simulink model "Current_Fed_DC_DC_Converter_Code_Equivalent_v4"  (R2020a)
settings: Solver=ode3  StartTime=0.0  StopTime=0.4  MaxStep=1e-5  MinStep=1e-7  RelTol=1e-6
InitFcn:
  | %Supply
  | V_supply = 415;
  | f_supply = 50;
  | 
  | %DC_Bus
  | C_filt = 220e-6
  | L_dc = 100e-6;
  | C_out = 560e-3;
  | 
  | %Transformer
  | P_TX = 10e3;
  | V_pri = 36;
  | V_sec = 1;
  | L_leak = 0;
  | R_leak = 0;
  | L_mag = inf;
  | R_mag = inf;
  | 
  | %Control
  | f_sw = 15e3;
  | tss_conv = 0.1;
  | V_ref = 1480;
  | Kp_V = 1;
  | Ki_V = 0.001;
  | I_ref = 2920;
  | Kp_I = 0.025;
  | Ki_I = 0.000001;
  | PS_max = 180;
  | Carr_offset = 1;
  | Carr_scale = 0.5;
  | Duty_scale = 0.01;
  | Duty_fix = 50;
  | Duty_max = 75;
  | Duty_min = 0;
  | f_chop = 1e3;
  | Duty_chop = 40;
  | 
  | %Harmonic_Correction
  | P_inj = 50;
  | f_inj = 50;
  | L_inj = 10e-6;
  | R_inj = 1;
  | Vpri_inj = 1;
  | Vsec_inj = 70;
  | Rleak_inj = 1e-3;
  | Lleak_inj = 12e-6;
  | R_inj = 0.1;
  | Rmag_inj = 1e-3;
  | Lmag_inj = 1e-3;
  | 
  | %Sensor
  | ADC_Res = 4096;
  | I_sense = 1/700;
  | V_sense = 1/50;
  | 
  | %Faults
  | OV_limit = 18.25;
  | UV_limit = 17.5;
  | OC_limit = 515;
  | UC_limit = 22;
  | ... (+3 lines)
libraries: powerlib x109, powerlib_meascontrol x30, simulink x5, slctrlblks x2
(part 3 of 3)

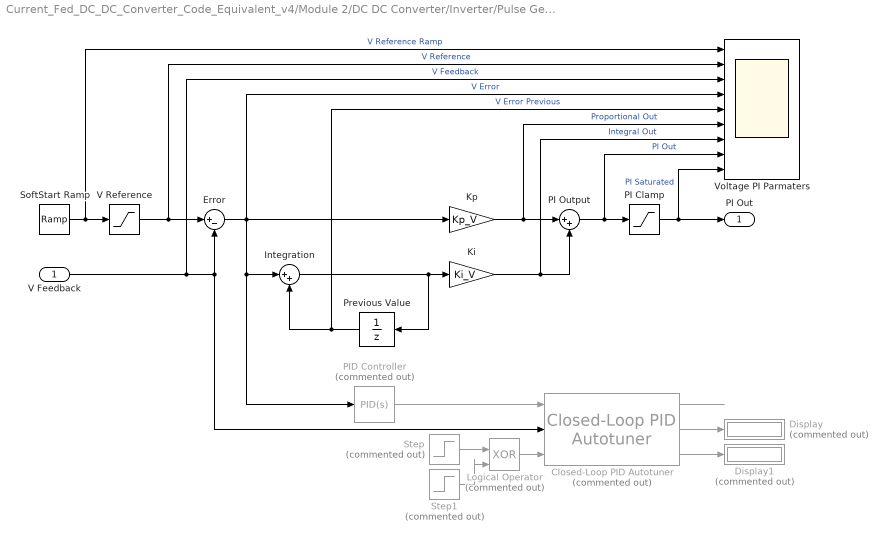
== system Current_Fed_DC_DC_Converter_Code_Equivalent_v4/Module 2/DC DC Converter/Inverter/Pulse Generator/Close Loop/Voltage Loop ==
  V Feedback : Inport
  Closed-Loop PID Autotuner : slctrlblks/Closed-Loop PID Autotuner  Commented=on  PIDType=PI  PIDForm=Parallel  TimeDomain=discrete-time  DiscreteTs=0.1  IntegratorFormula=Forward Euler  FilterFormula=Forward Euler  ContinuousTs=0.02  Bandwidth=1  UseExternalWC=off  TargetPM=60  UseExternalPM=off  UseExternalAchievedPM=off  PlantType=Stable  PlantSign=Positive  AmpSine=1  UseExternalAmpSine=off  UseExternalFRD=off  UseExternalU0=off  UseCompanion=off  NotDeployTuningModule=off  UsePLCCoder=off  OutputMode=control action + perturbation  BlockDataType=double  UseConnectedPID=on  blockpath=[]  tunedP=0  tunedI=0  tunedD=0  tunedN=100  tunedPM=0  EstimationWindowSize=3  UseExternalTuningParams=off  OutputChoice=VariantCandD
      settings: SourceProductBaseCode=SD
  Display : Display  Commented=on
  Display1 : Display  Commented=on
  Error : Sum  Inputs=|+-
  Integration : Sum  Inputs=|++
  Ki : Gain  Gain=Ki_V
  Kp : Gain  Gain=Kp_V
  Logical Operator : Logic  Commented=on  Operator=XOR  IconShape=distinctive  AllPortsSameDT=off  OutDataTypeStr=boolean
  PI Clamp : Saturate  UpperLimit=I_ref  LowerLimit=0
  PI Output : Sum  Inputs=|++
  PID Controller : simulink/Continuous/PID Controller  Commented=on  Controller=PID  Form=Parallel  TimeDomain=Continuous-time  UseExternalTs=off  SampleTime=-1  IntegratorMethod=Forward Euler  FilterMethod=Forward Euler  ControllerParametersSource=internal  P=1  I=1  D=0  UseFilter=on  N=100  TunerSelectOption=Transfer Function Based (PID Tuner App)  InitialConditionSource=internal  InitialConditionForIntegrator=0  InitialConditionForFilter=0  DifferentiatorICPrevScaledInput=0  ExternalReset=none  TrackingMode=off  Kt=1  LimitOutput=off  UpperSaturationLimit=inf  LowerSaturationLimit=-inf  LinearizeAsGain=on  AntiWindupMode=none  Kb=1  POutMin=[]  POutMax=[]  IOutMin=[]  IOutMax=[]  DOutMin=[]  DOutMax=[]  NOutMin=[]  NOutMax=[]  SumOutMin=[]  SumOutMax=[]  SaturationOutMin=[]  SaturationOutMax=[]  PParamMin=[]  PParamMax=[]  IParamMin=[]  IParamMax=[]  DParamMin=[]  DParamMax=[]  NParamMin=[]  NParamMax=[]  KbParamMin=[]  KbParamMax=[]  KtParamMin=[]  KtParamMax=[]  KbOutMin=[]  KbOutMax=[]  KtOutMin=[]  KtOutMax=[]  IntegratorOutMin=[]  IntegratorOutMax=[]  FilterOutMin=[]  FilterOutMax=[]  SumI1OutMin=[]  SumI1OutMax=[]  SumI2OutMin=[]  SumI2OutMax=[]  SumI3OutMin=[]  SumI3OutMax=[]  SumI4OutMin=[]  SumI4OutMax=[]  SumDOutMin=[]  SumDOutMax=[]  DifferentiatorOutMin=[]  DifferentiatorOutMax=[]  FilterDiffOutCoefMin=[]  FilterDiffOutCoefMax=[]  ReciprocalOutMin=[]  ReciprocalOutMax=[]  SumDenOutMin=[]  SumDenOutMax=[]  SumNumOutMin=[]  SumNumOutMax=[]  DivideOutMin=[]  DivideOutMax=[]  UdiffTsProdOutMin=[]  UdiffTsProdOutMax=[]  NTsProdOutMin=[]  NTsProdOutMax=[]  UintegralTsProdOutMin=[]  UintegralTsProdOutMax=[]  UngainTsProdOutMin=[]  UngainTsProdOutMax=[]  IntegratorContinuousStateAttributes=''  IntegratorStateMustResolveToSignalObject=off  IntegratorRTWStateStorageClass=Auto  FilterContinuousStateAttributes=''  FilterStateMustResolveToSignalObject=off  FilterRTWStateStorageClass=Auto  ParallelPVariant=InternalParameters  IdealPVariant=Disabled  IVariant=InternalParameters  DVariant=InternalParameters  IntegratorVariant=Continuous  SatVariant=Disabled  AWVariant=Passthrough  PCopyVariant=Disabled  TRVariant=Disabled  FdbkBlocksVariant=Forward  IdealPFdbkVariant=Disabled  SatFdbkVariant=Disabled  DerivativeFilterVariant=ContFilter  NVariant=InternalParameters  NCopyVariant=Disabled  FilterICVariant=InternalICsFilter  IntegratorICVariant=InternalICs  ExternalResetVariant=Disabled  TRSumVariant=Passthrough  SumFdbkVariant=Disabled  SumVariant=Sum_PID  TsampFilterVariant=InternalTs  TsampNgainVariant=Passthrough  TsampIntegralVariant=Passthrough
  Previous Value : UnitDelay  SampleTime=-1  HasFrameUpgradeWarning=on
  SoftStart Ramp : simulink/Sources/Ramp  slope=V_ref/tss_conv  start=0  InitialOutput=0
  Step : Step  Commented=on  Time=0  SampleTime=0
  Step1 : Step  Commented=on  SampleTime=0
  V Reference : Saturate  UpperLimit=V_ref  LowerLimit=0
  Voltage PI Parmaters : Scope  NumInputPorts=9
  PI Out : Outport
  wires:
  Step1/1 -> Logical Operator/2
  Step/1 -> Logical Operator/1
  Logical Operator/1 -> Closed-Loop PID Autotuner/3
  Closed-Loop PID Autotuner/3 -> Display1/1
  Closed-Loop PID Autotuner/2 -> Display/1
  Closed-Loop PID Autotuner/1 -> ?
  PID Controller/1 -> Closed-Loop PID Autotuner/1
  PI Clamp/1 -> Voltage PI Parmaters/9, PI Out/1  "PI Saturated"
  SoftStart Ramp/1 -> Voltage PI Parmaters/1, V Reference/1  "V Reference Ramp"
  V Reference/1 -> Voltage PI Parmaters/2, Error/1  "V Reference"
  Ki/1 -> Voltage PI Parmaters/7, PI Output/2  "Integral Out"
  Error/1 -> Integration/1, PID Controller/1, Voltage PI Parmaters/4, Kp/1  "V Error"
  PI Output/1 -> Voltage PI Parmaters/8, PI Clamp/1  "PI Out"
  V Feedback/1 -> Voltage PI Parmaters/3, Error/2, Closed-Loop PID Autotuner/2  "V Feedback"
  Kp/1 -> Voltage PI Parmaters/6, PI Output/1  "Proportional Out"
  Previous Value/1 -> Integration/2, Voltage PI Parmaters/5  "V Error Previous"
  Integration/1 -> Ki/1, Previous Value/1

== system Current_Fed_DC_DC_Converter_Code_Equivalent_v4/Module 3/DC DC Converter/Inverter/Pulse Generator/Close Loop/Current Loop ==
  I Reference : Inport
  I Feedback : Inport  Port=2
  Current PI Parmaters : Scope  NumInputPorts=8
  Error : Sum  Inputs=|+-
  Integrate : Sum  Inputs=|++
  Ki : Gain  Gain=Ki_I
  Kp : Gain  Gain=Kp_I
  PI : Sum  Inputs=|++
  PI Clamp : Saturate  UpperLimit=Duty_max  LowerLimit=Duty_min
  Previous Value : UnitDelay  SampleTime=-1  HasFrameUpgradeWarning=on
  Reference Clamp : Saturate  UpperLimit=I_ref  LowerLimit=0
  PI Out : Outport
  wires:
  Reference Clamp/1 -> Error/1, Current PI Parmaters/1  "PI Saturated"
  PI/1 -> Current PI Parmaters/7, PI Clamp/1  "Duty Cycle Shift"
  PI Clamp/1 -> Current PI Parmaters/8, PI Out/1  "Duty Cycle Clamped"
  I Feedback/1 -> Current PI Parmaters/2, Error/2  "I Feedback"
  I Reference/1 -> Reference Clamp/1  "I Reference"
  Error/1 -> Integrate/1, Current PI Parmaters/3, Kp/1  "I Error"
  Integrate/1 -> Previous Value/1, Ki/1
  Ki/1 -> Current PI Parmaters/6, PI/2  "Integral Out"
  Kp/1 -> Current PI Parmaters/5, PI/1  "Proportional Out"
  Previous Value/1 -> Integrate/2, Current PI Parmaters/4  "I Error Previous"

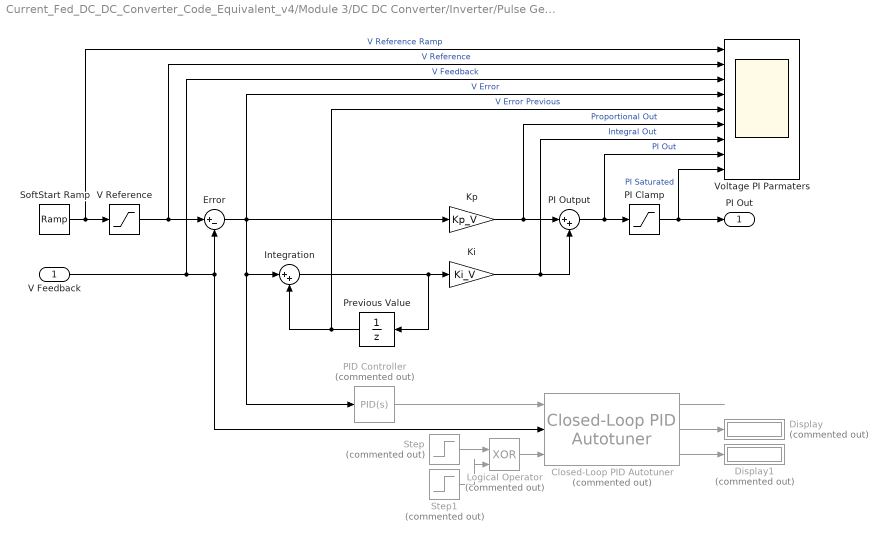
== system Current_Fed_DC_DC_Converter_Code_Equivalent_v4/Module 3/DC DC Converter/Inverter/Pulse Generator/Close Loop/Voltage Loop ==
  V Feedback : Inport
  Closed-Loop PID Autotuner : slctrlblks/Closed-Loop PID Autotuner  Commented=on  PIDType=PI  PIDForm=Parallel  TimeDomain=discrete-time  DiscreteTs=0.1  IntegratorFormula=Forward Euler  FilterFormula=Forward Euler  ContinuousTs=0.02  Bandwidth=1  UseExternalWC=off  TargetPM=60  UseExternalPM=off  UseExternalAchievedPM=off  PlantType=Stable  PlantSign=Positive  AmpSine=1  UseExternalAmpSine=off  UseExternalFRD=off  UseExternalU0=off  UseCompanion=off  NotDeployTuningModule=off  UsePLCCoder=off  OutputMode=control action + perturbation  BlockDataType=double  UseConnectedPID=on  blockpath=[]  tunedP=0  tunedI=0  tunedD=0  tunedN=100  tunedPM=0  EstimationWindowSize=3  UseExternalTuningParams=off  OutputChoice=VariantCandD
      settings: SourceProductBaseCode=SD
  Display : Display  Commented=on
  Display1 : Display  Commented=on
  Error : Sum  Inputs=|+-
  Integration : Sum  Inputs=|++
  Ki : Gain  Gain=Ki_V
  Kp : Gain  Gain=Kp_V
  Logical Operator : Logic  Commented=on  Operator=XOR  IconShape=distinctive  AllPortsSameDT=off  OutDataTypeStr=boolean
  PI Clamp : Saturate  UpperLimit=I_ref  LowerLimit=0
  PI Output : Sum  Inputs=|++
  PID Controller : simulink/Continuous/PID Controller  Commented=on  Controller=PID  Form=Parallel  TimeDomain=Continuous-time  UseExternalTs=off  SampleTime=-1  IntegratorMethod=Forward Euler  FilterMethod=Forward Euler  ControllerParametersSource=internal  P=1  I=1  D=0  UseFilter=on  N=100  TunerSelectOption=Transfer Function Based (PID Tuner App)  InitialConditionSource=internal  InitialConditionForIntegrator=0  InitialConditionForFilter=0  DifferentiatorICPrevScaledInput=0  ExternalReset=none  TrackingMode=off  Kt=1  LimitOutput=off  UpperSaturationLimit=inf  LowerSaturationLimit=-inf  LinearizeAsGain=on  AntiWindupMode=none  Kb=1  POutMin=[]  POutMax=[]  IOutMin=[]  IOutMax=[]  DOutMin=[]  DOutMax=[]  NOutMin=[]  NOutMax=[]  SumOutMin=[]  SumOutMax=[]  SaturationOutMin=[]  SaturationOutMax=[]  PParamMin=[]  PParamMax=[]  IParamMin=[]  IParamMax=[]  DParamMin=[]  DParamMax=[]  NParamMin=[]  NParamMax=[]  KbParamMin=[]  KbParamMax=[]  KtParamMin=[]  KtParamMax=[]  KbOutMin=[]  KbOutMax=[]  KtOutMin=[]  KtOutMax=[]  IntegratorOutMin=[]  IntegratorOutMax=[]  FilterOutMin=[]  FilterOutMax=[]  SumI1OutMin=[]  SumI1OutMax=[]  SumI2OutMin=[]  SumI2OutMax=[]  SumI3OutMin=[]  SumI3OutMax=[]  SumI4OutMin=[]  SumI4OutMax=[]  SumDOutMin=[]  SumDOutMax=[]  DifferentiatorOutMin=[]  DifferentiatorOutMax=[]  FilterDiffOutCoefMin=[]  FilterDiffOutCoefMax=[]  ReciprocalOutMin=[]  ReciprocalOutMax=[]  SumDenOutMin=[]  SumDenOutMax=[]  SumNumOutMin=[]  SumNumOutMax=[]  DivideOutMin=[]  DivideOutMax=[]  UdiffTsProdOutMin=[]  UdiffTsProdOutMax=[]  NTsProdOutMin=[]  NTsProdOutMax=[]  UintegralTsProdOutMin=[]  UintegralTsProdOutMax=[]  UngainTsProdOutMin=[]  UngainTsProdOutMax=[]  IntegratorContinuousStateAttributes=''  IntegratorStateMustResolveToSignalObject=off  IntegratorRTWStateStorageClass=Auto  FilterContinuousStateAttributes=''  FilterStateMustResolveToSignalObject=off  FilterRTWStateStorageClass=Auto  ParallelPVariant=InternalParameters  IdealPVariant=Disabled  IVariant=InternalParameters  DVariant=InternalParameters  IntegratorVariant=Continuous  SatVariant=Disabled  AWVariant=Passthrough  PCopyVariant=Disabled  TRVariant=Disabled  FdbkBlocksVariant=Forward  IdealPFdbkVariant=Disabled  SatFdbkVariant=Disabled  DerivativeFilterVariant=ContFilter  NVariant=InternalParameters  NCopyVariant=Disabled  FilterICVariant=InternalICsFilter  IntegratorICVariant=InternalICs  ExternalResetVariant=Disabled  TRSumVariant=Passthrough  SumFdbkVariant=Disabled  SumVariant=Sum_PID  TsampFilterVariant=InternalTs  TsampNgainVariant=Passthrough  TsampIntegralVariant=Passthrough
  Previous Value : UnitDelay  SampleTime=-1  HasFrameUpgradeWarning=on
  SoftStart Ramp : simulink/Sources/Ramp  slope=V_ref/tss_conv  start=0  InitialOutput=0
  Step : Step  Commented=on  Time=0  SampleTime=0
  Step1 : Step  Commented=on  SampleTime=0
  V Reference : Saturate  UpperLimit=V_ref  LowerLimit=0
  Voltage PI Parmaters : Scope  NumInputPorts=9
  PI Out : Outport
  wires:
  Step1/1 -> Logical Operator/2
  Step/1 -> Logical Operator/1
  Logical Operator/1 -> Closed-Loop PID Autotuner/3
  Closed-Loop PID Autotuner/3 -> Display1/1
  Closed-Loop PID Autotuner/2 -> Display/1
  Closed-Loop PID Autotuner/1 -> ?
  PID Controller/1 -> Closed-Loop PID Autotuner/1
  PI Clamp/1 -> Voltage PI Parmaters/9, PI Out/1  "PI Saturated"
  SoftStart Ramp/1 -> Voltage PI Parmaters/1, V Reference/1  "V Reference Ramp"
  V Reference/1 -> Voltage PI Parmaters/2, Error/1  "V Reference"
  Ki/1 -> Voltage PI Parmaters/7, PI Output/2  "Integral Out"
  Error/1 -> Integration/1, PID Controller/1, Voltage PI Parmaters/4, Kp/1  "V Error"
  PI Output/1 -> Voltage PI Parmaters/8, PI Clamp/1  "PI Out"
  V Feedback/1 -> Voltage PI Parmaters/3, Error/2, Closed-Loop PID Autotuner/2  "V Feedback"
  Kp/1 -> Voltage PI Parmaters/6, PI Output/1  "Proportional Out"
  Previous Value/1 -> Integration/2, Voltage PI Parmaters/5  "V Error Previous"
  Integration/1 -> Ki/1, Previous Value/1
